simulink model "observateur2"  (R2020a)
settings: Solver=VariableStepAuto  StartTime=0.0  StopTime=100  RelTol=1e-3
undefined symbols (not defined in the file): a, b, L, lambda
settings Model: Creator=lenovo  LastModifiedBy=lenovo

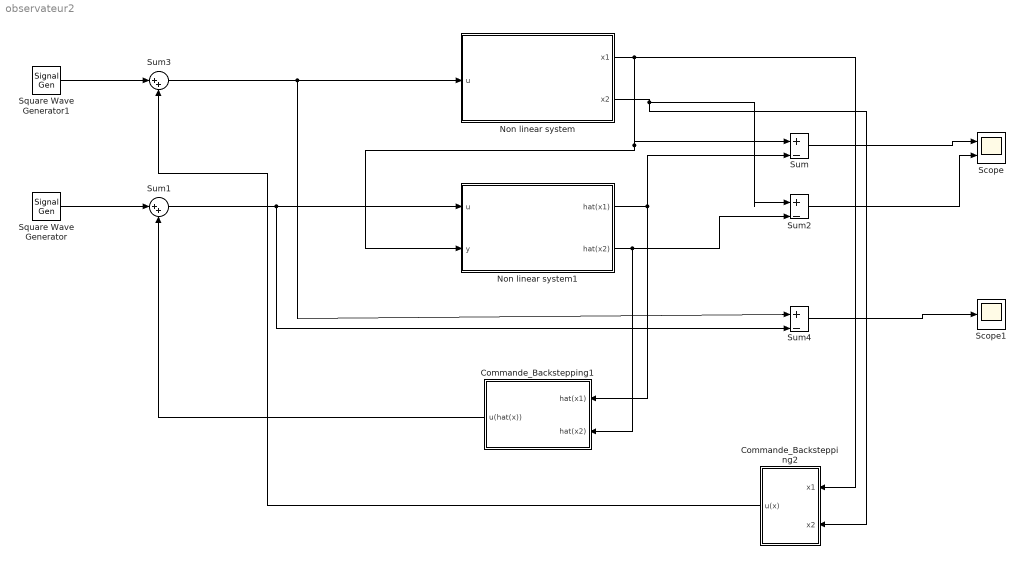
== system observateur2 ==
  Commande_Backstepping1 : Subsystem
  Commande_Backstepping2 : Subsystem
  Non linear system : Subsystem
  Non linear system1 : Subsystem
  Scope : Scope  NumInputPorts=2
  Scope1 : Scope
  Square Wave Generator : SignalGenerator  WaveForm=square  Units=rad/sec
  Square Wave Generator1 : SignalGenerator  WaveForm=square  Units=rad/sec
  Sum : Sum  Inputs=|+-
  Sum1 : Sum  Inputs=|++
  Sum2 : Sum  Inputs=|+-
  Sum3 : Sum  Inputs=|++
  Sum4 : Sum  Inputs=|+-
  wires:
  Non linear system1/1(hat(x1)) -> Commande_Backstepping1/1(hat(x1)), Sum/2
  Square Wave Generator/1 -> Sum1/1
  Sum/1 -> Scope/1
  Sum2/1 -> Scope/2
  Non linear system1/2(hat(x2)) -> Commande_Backstepping1/2(hat(x2)), Sum2/2
  Non linear system/2(x2) -> Sum2/1, Commande_Backstepping2/2(x2)
  Non linear system/1(x1) -> Commande_Backstepping2/1(x1), Non linear system1/2(y), Sum/1
  Square Wave Generator1/1 -> Sum3/1
  Commande_Backstepping1/1(u(hat(x))) -> Sum1/2
  Commande_Backstepping2/1(u(x)) -> Sum3/2
  Sum4/1 -> Scope1/1
  Sum1/1 -> Sum4/2, Non linear system1/1(u)
  Sum3/1 -> Sum4/1, Non linear system/1(u)

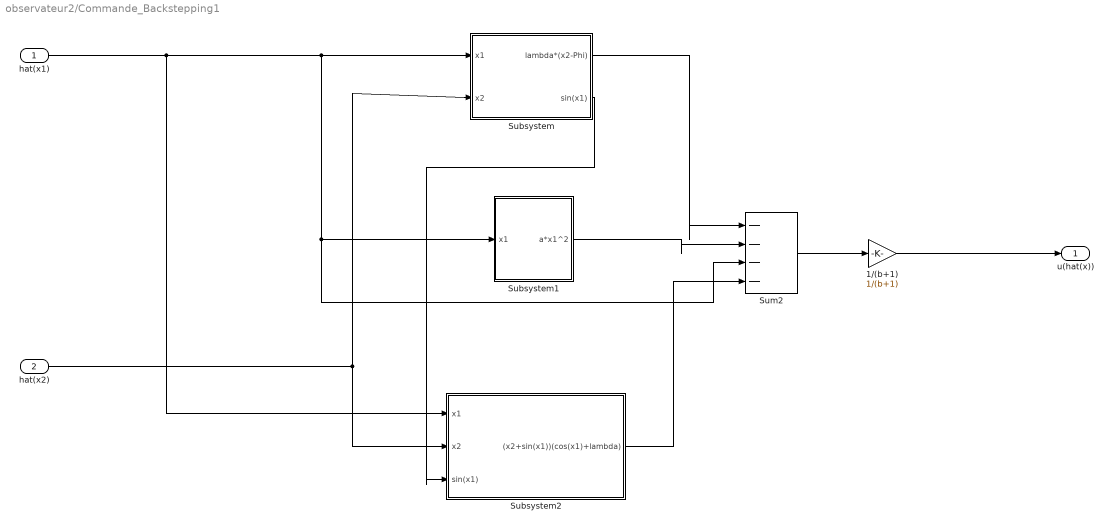
== system observateur2/Commande_Backstepping1 ==
  hat(x1) : Inport
  hat(x2) : Inport  Port=2
  1/(b+1) : Gain  Gain=1/(b+1)
  Subsystem : Subsystem
  Subsystem1 : Subsystem
  Subsystem2 : Subsystem
  Sum2 : Sum  Inputs=|----
  u(hat(x)) : Outport
  wires:
  hat(x1)/1 -> Subsystem2/1("x1 "), Subsystem/1(x1), Sum2/3, Subsystem1/1("x1 ")
  hat(x2)/1 -> Subsystem2/2(x2), Subsystem/2(x2)
  Sum2/1 -> 1/(b+1)/1
  1/(b+1)/1 -> u(hat(x))/1
  Subsystem/1(lambda*(x2-Phi)) -> Sum2/1
  Subsystem1/1(a*x1^2) -> Sum2/2
  Subsystem/2(sin(x1)) -> Subsystem2/3(sin(x1))
  Subsystem2/1((x2+sin(x1))(cos(x1)+lambda)) -> Sum2/4

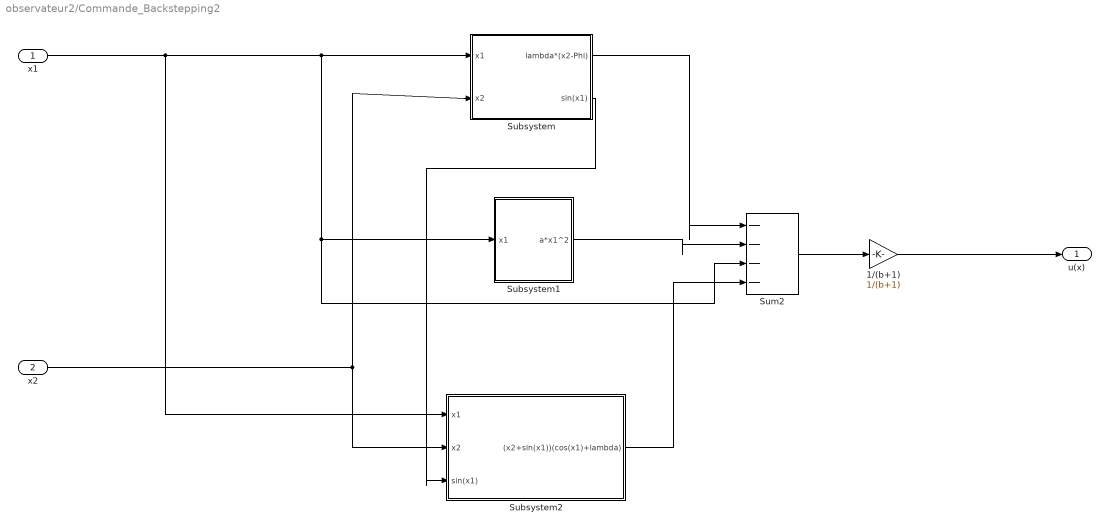
== system observateur2/Commande_Backstepping2 ==
  x1 : Inport
  x2 : Inport  Port=2
  1/(b+1) : Gain  Gain=1/(b+1)
  Subsystem : Subsystem
  Subsystem1 : Subsystem
  Subsystem2 : Subsystem
  Sum2 : Sum  Inputs=|----
  u(x) : Outport
  wires:
  x1/1 -> Subsystem2/1("x1 "), Subsystem/1(x1), Sum2/3, Subsystem1/1("x1 ")
  x2/1 -> Subsystem2/2(x2), Subsystem/2(x2)
  Sum2/1 -> 1/(b+1)/1
  1/(b+1)/1 -> u(x)/1
  Subsystem/1(lambda*(x2-Phi)) -> Sum2/1
  Subsystem1/1(a*x1^2) -> Sum2/2
  Subsystem/2(sin(x1)) -> Subsystem2/3(sin(x1))
  Subsystem2/1((x2+sin(x1))(cos(x1)+lambda)) -> Sum2/4

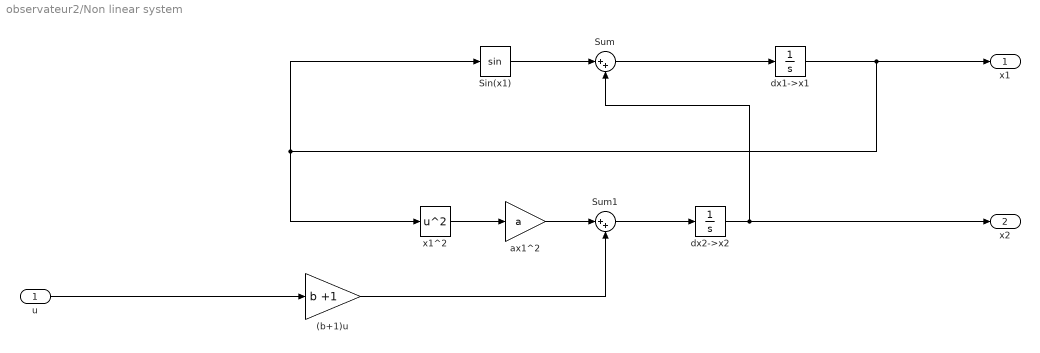
== system observateur2/Non linear system ==
  u : Inport
  (b+1)u : Gain  Gain=b +1
  Sin(x1) : Trigonometry
  Sum : Sum  Inputs=|++
  Sum1 : Sum  Inputs=|++
  ax1^2 : Gain  Gain=a
  dx1->x1 : Integrator
  dx2->x2 : Integrator
  x1^2 : Math  Operator=square  SaturateOnIntegerOverflow=on
  x1 : Outport
  x2 : Outport  Port=2
  wires:
  (b+1)u/1 -> Sum1/2
  dx2->x2/1 -> x2/1, Sum/2
  u/1 -> (b+1)u/1
  ax1^2/1 -> Sum1/1
  dx1->x1/1 -> Sin(x1)/1, x1^2/1, x1/1
  Sin(x1)/1 -> Sum/1
  x1^2/1 -> ax1^2/1
  Sum1/1 -> dx2->x2/1
  Sum/1 -> dx1->x1/1

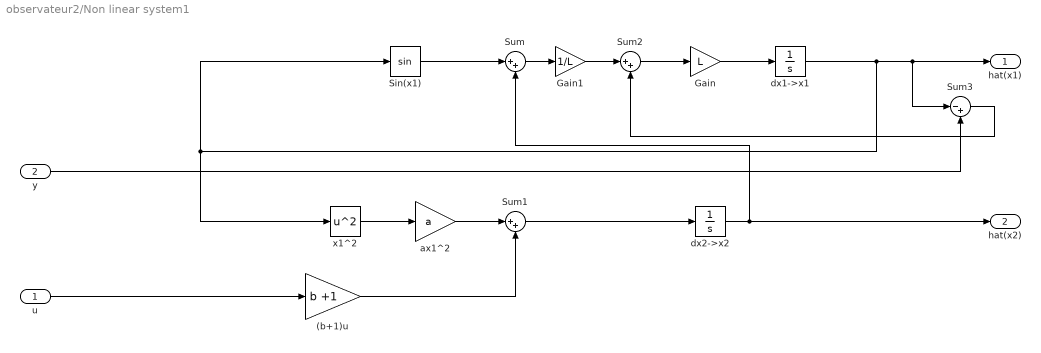
== system observateur2/Non linear system1 ==
  u : Inport
  y : Inport  Port=2
  (b+1)u : Gain  Gain=b +1
  Gain : Gain  Gain=L
  Gain1 : Gain  Gain=1/L
  Sin(x1) : Trigonometry
  Sum : Sum  Inputs=|++
  Sum1 : Sum  Inputs=|++
  Sum2 : Sum  Inputs=|++
  Sum3 : Sum  Inputs=|-+
  ax1^2 : Gain  Gain=a
  dx1->x1 : Integrator
  dx2->x2 : Integrator  InitialCondition=1
  x1^2 : Math  Operator=square  SaturateOnIntegerOverflow=on
  hat(x1) : Outport
  hat(x2) : Outport  Port=2
  wires:
  (b+1)u/1 -> Sum1/2
  dx2->x2/1 -> hat(x2)/1, Sum/2
  u/1 -> (b+1)u/1
  ax1^2/1 -> Sum1/1
  dx1->x1/1 -> Sin(x1)/1, x1^2/1, Sum3/1, hat(x1)/1
  Sin(x1)/1 -> Sum/1
  x1^2/1 -> ax1^2/1
  Sum1/1 -> dx2->x2/1
  Sum/1 -> Gain1/1
  y/1 -> Sum3/2
  Sum3/1 -> Sum2/2
  Sum2/1 -> Gain/1
  Gain/1 -> dx1->x1/1
  Gain1/1 -> Sum2/1

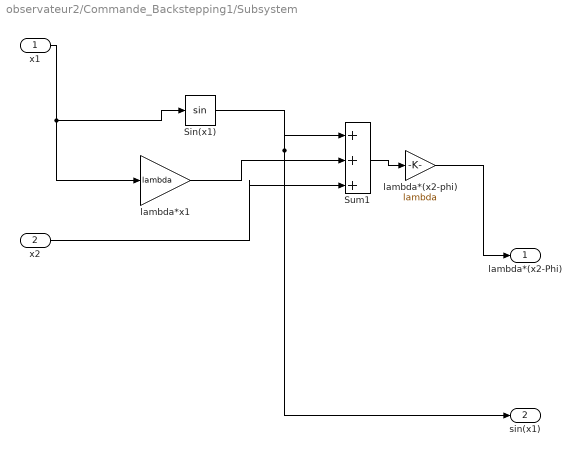
== system observateur2/Commande_Backstepping1/Subsystem ==
  x1 : Inport
  x2 : Inport  Port=2
  Sin(x1) : Trigonometry
  Sum1 : Sum  Inputs=|+++
  lambda*(x2-phi) : Gain  Gain=lambda
  lambda*x1 : Gain  Gain=lambda
  lambda*(x2-Phi) : Outport
  sin(x1) : Outport  Port=2
  wires:
  x1/1 -> Sin(x1)/1, lambda*x1/1
  Sin(x1)/1 -> sin(x1)/1, Sum1/1
  Sum1/1 -> lambda*(x2-phi)/1
  x2/1 -> Sum1/3
  lambda*x1/1 -> Sum1/2
  lambda*(x2-phi)/1 -> lambda*(x2-Phi)/1

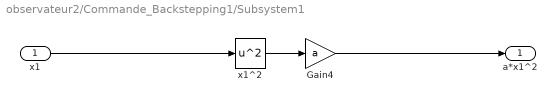
== system observateur2/Commande_Backstepping1/Subsystem1 ==
  "x1 " : Inport
  Gain4 : Gain  Gain=a
  x1^2 : Math  Operator=square  SaturateOnIntegerOverflow=on
  a*x1^2 : Outport
  wires:
  x1^2/1 -> Gain4/1
  Gain4/1 -> a*x1^2/1
  "x1 "/1 -> x1^2/1

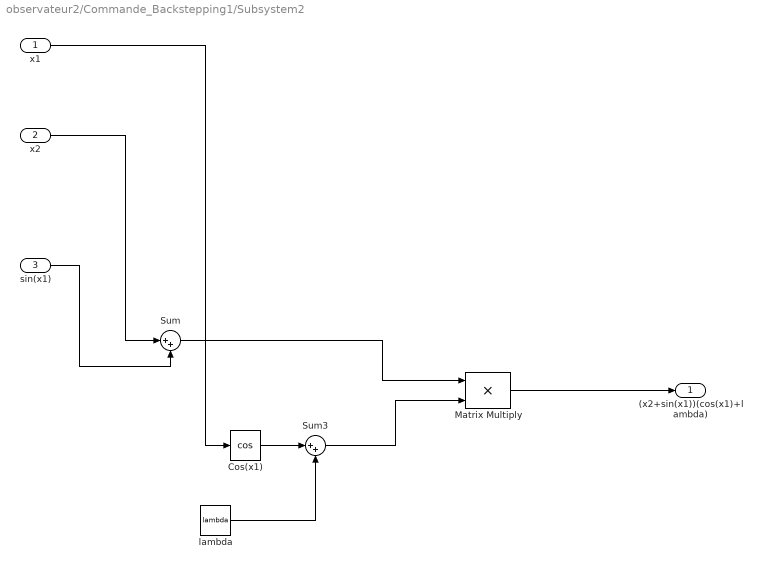
== system observateur2/Commande_Backstepping1/Subsystem2 ==
  "x1 " : Inport
  x2 : Inport  Port=2
  sin(x1) : Inport  Port=3
  Cos(x1) : Trigonometry  Operator=cos
  Matrix Multiply : Product
  Sum : Sum  Inputs=|++
  Sum3 : Sum  Inputs=|++
  lambda : Constant  Value=lambda  OutDataTypeStr=Inherit: Inherit via back propagation
  (x2+sin(x1))(cos(x1)+lambda) : Outport
  wires:
  Cos(x1)/1 -> Sum3/1
  sin(x1)/1 -> Sum/2
  lambda/1 -> Sum3/2
  x2/1 -> Sum/1
  Matrix Multiply/1 -> (x2+sin(x1))(cos(x1)+lambda)/1
  Sum/1 -> Matrix Multiply/1
  Sum3/1 -> Matrix Multiply/2
  "x1 "/1 -> Cos(x1)/1

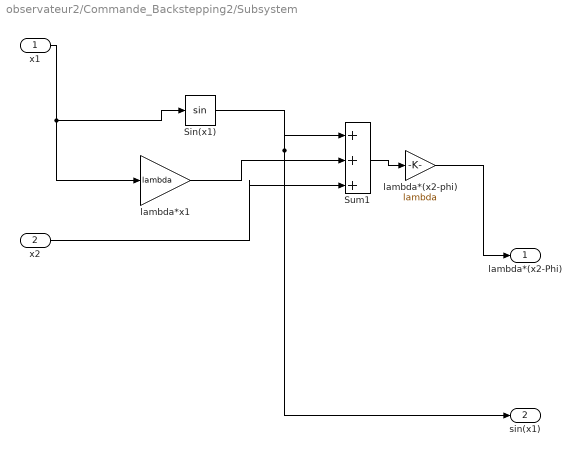
== system observateur2/Commande_Backstepping2/Subsystem ==
  x1 : Inport
  x2 : Inport  Port=2
  Sin(x1) : Trigonometry
  Sum1 : Sum  Inputs=|+++
  lambda*(x2-phi) : Gain  Gain=lambda
  lambda*x1 : Gain  Gain=lambda
  lambda*(x2-Phi) : Outport
  sin(x1) : Outport  Port=2
  wires:
  x1/1 -> Sin(x1)/1, lambda*x1/1
  Sin(x1)/1 -> sin(x1)/1, Sum1/1
  Sum1/1 -> lambda*(x2-phi)/1
  x2/1 -> Sum1/3
  lambda*x1/1 -> Sum1/2
  lambda*(x2-phi)/1 -> lambda*(x2-Phi)/1

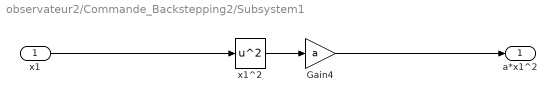
== system observateur2/Commande_Backstepping2/Subsystem1 ==
  "x1 " : Inport
  Gain4 : Gain  Gain=a
  x1^2 : Math  Operator=square  SaturateOnIntegerOverflow=on
  a*x1^2 : Outport
  wires:
  x1^2/1 -> Gain4/1
  Gain4/1 -> a*x1^2/1
  "x1 "/1 -> x1^2/1

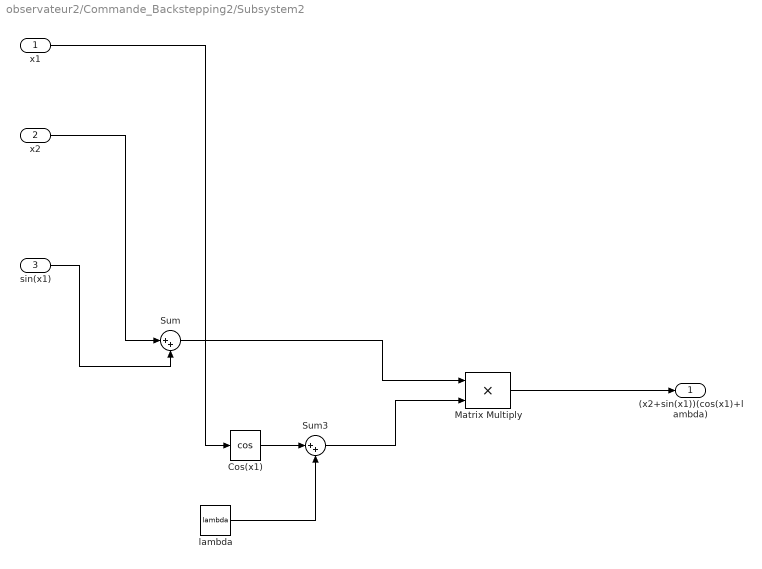
== system observateur2/Commande_Backstepping2/Subsystem2 ==
  "x1 " : Inport
  x2 : Inport  Port=2
  sin(x1) : Inport  Port=3
  Cos(x1) : Trigonometry  Operator=cos
  Matrix Multiply : Product
  Sum : Sum  Inputs=|++
  Sum3 : Sum  Inputs=|++
  lambda : Constant  Value=lambda  OutDataTypeStr=Inherit: Inherit via back propagation
  (x2+sin(x1))(cos(x1)+lambda) : Outport
  wires:
  Cos(x1)/1 -> Sum3/1
  sin(x1)/1 -> Sum/2
  lambda/1 -> Sum3/2
  x2/1 -> Sum/1
  Matrix Multiply/1 -> (x2+sin(x1))(cos(x1)+lambda)/1
  Sum/1 -> Matrix Multiply/1
  Sum3/1 -> Matrix Multiply/2
  "x1 "/1 -> Cos(x1)/1
